simulink model "seno"  (R2022a)
settings: Solver=ode4  StartTime=0.0  StopTime=10.0  FixedStep=0.01  RelTol=1e-3
settings Model: Creator=leonardonavacastellanos  LastModifiedBy=leonardonavacastellanos

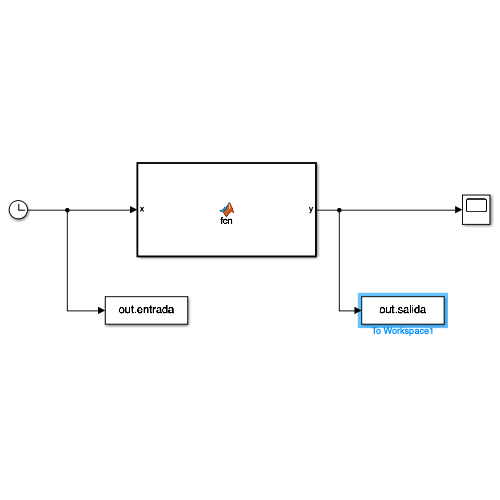
[thumbnail: Simulink's stored preview of the top-level diagram]
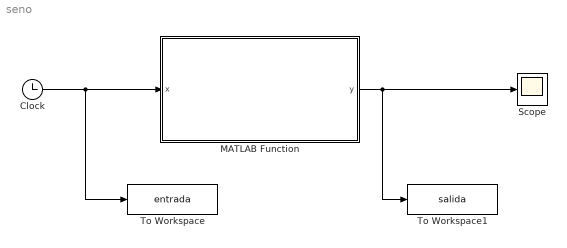
== system seno ==
  Clock : Clock
  MATLAB Function : MATLAB Function  TreatAsAtomicUnit=on
  Scope : Scope
  To Workspace : ToWorkspace  VariableName=entrada  SampleTime=-1
      settings: Save2DSignal=2-D array (concatenate along first dimension)
  To Workspace1 : ToWorkspace  VariableName=salida  SampleTime=-1
      settings: Save2DSignal=2-D array (concatenate along first dimension)
  wires:
  Clock/1 -> MATLAB Function/1(x), To Workspace/1
  MATLAB Function/1(y) -> Scope/1, To Workspace1/1

== matlab function seno/MATLAB Function ==
  data: x input; y output
function y = fcn(x)

y = sin(x);
